simulink model "control_core"  (R2022b)
settings: Solver=FixedStepAuto  StartTime=0.0  StopTime=60  FixedStep=.01  RelTol=1e-3
undefined symbols (not defined in the file): CdProp, Ct, g, Ixx, Iyy, Izz, larm, mass
libraries: slpidlib x6, sharedtransform x2, simulink x2, aerolibutil x2, shared6dof x1, aerolibfltsims x1, vrlib x1
(part 2 of 2)

== matlab function control_core/Controllers/Motor Mixing/MATLAB Function ==
  data: controlMatInv output; Ct parameter; larm parameter; CdProp parameter
function controlMatInv = calc_motor_speed(Ct,...
larm, CdProp)
% u1 = force;
% u2 = torques(1);
% u3 = torques(2);
% u4 = torques(3);


K = Ct;
L = larm;
C = CdProp;

% invControlMat = -[(C*u2 + C*u3 + C*L*u1 + K*L*u4)/(4*C*K*L);
%  (C*u2 - C*u3 - C*L*u1 + K*L*u4)/(4*C*K*L);
%  (C*u2 + C*u3 - C*L*u1 - K*L*u4)/(4*C*K*L);
% -(C*u2 - C*u3 + C*L*u1 - K*L*u4)/(4*C*K*L)];

invControlMat = [-1/(4*K), -1/(4*K*L), -1/(4*K*L), -1/(4*C);
                -1/(4*K),  1/(4*K*L), -1/(4*K*L),  1/(4*C);
                -1/(4*K),  1/(4*K*L),  1/(4*K*L), -1/(4*C);
                -1/(4*K), -1/(4*K*L),  1/(4*K*L),  1/(4*C)];
controlMatInv = invControlMat;
